simulink model "ex01_model"  (R2023a)
settings: Solver=FixedStepDiscrete  StartTime=0.0  StopTime=20*Ts  RelTol=1e-3
values from neighbouring files (symbols this model uses):
  Fc = 1e3    (= 1000)    [ex00.m]    (also in ex01_config.m; ex02_config.m)
  L = 2    [ex01_config.m]    (also in ex02_config.m = 3)
  Ts = 1/Fs    (= 6.25e-05)    [ex00.m]    (also in ex01_config.m; ex02_config.m)
libraries: dspsrcs4 x1, dspsigops x1
settings Model: Creator=daniele  LastModifiedBy=daniele
settings SolverCC: AlgebraicLoopSolver=TrustRegion
settings DataIOCC: ReturnWorkspaceOutputs=off
settings DebuggingCC: UnconnectedInputMsg=warning  UnconnectedOutputMsg=warning  UnconnectedLineMsg=warning  ArithmeticOperatorsInVariantConditions=warning
settings ModelReferenceCC: EnableRefExpFcnMdlSchedulingChecks=on
settings SFSimCC: CustomCodeUndefinedFunction=UseInterfaceOnly

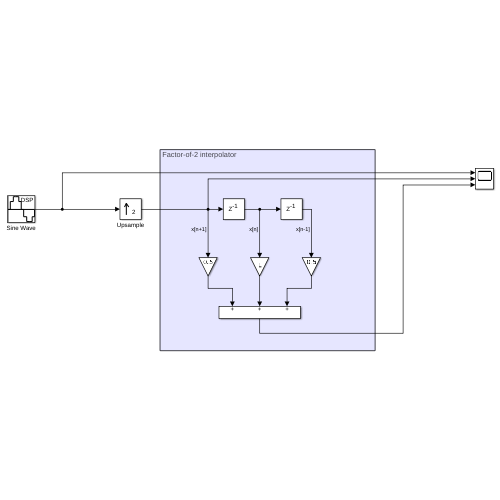
[thumbnail: Simulink's stored preview of the top-level diagram]
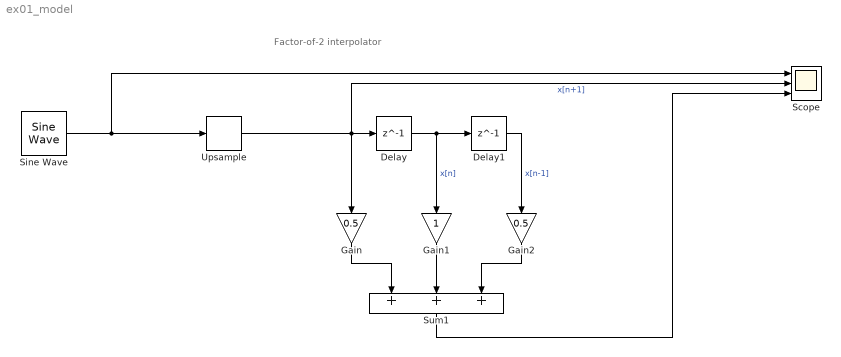
== system ex01_model ==
  note: Factor-of-2 interpolator
  Delay : Delay  DelayLength=1
  Delay1 : Delay  DelayLength=1
  Gain : Gain  Gain=0.5
  Gain1 : Gain
  Gain2 : Gain  Gain=0.5
  Scope : Scope  NumInputPorts=3
  Sine Wave : dspsrcs4/Sine Wave  Amplitude=1  Frequency=Fc  Phase=0  SampleMode=Discrete  OutComplex=Real  CompMethod=Trigonometric fcn  TableSize=Speed  SampleTime=Ts  SamplesPerFrame=1  ResetState=Restart at time zero  OutputFrames=off  dataType=double  wordLen=16  udDataType=sfix(16)  fracBitsMode=Best precision  numFracBits=15  OutDataTypeStr=double  LastOutDataTypeStr=double
  Sum1 : Sum  Inputs=+++
  Upsample : dspsigops/Upsample  FactorSource=Dialog parameter  N=L  Nmax=16  phase=0  RateOptions=Allow multirate processing  ic=0  mode=Unused parameter value
      settings: LibrarySourceBlock=dsphdlsupportsigops/Upsample
  wires:
  Sine Wave/1 -> Upsample/1, Scope/1
  Delay/1 -> Gain1/1, Delay1/1  "x[n]"
  Delay1/1 -> Gain2/1  "x[n-1]"
  Upsample/1 -> Gain/1, Scope/2, Delay/1  "x[n+1]"
  Sum1/1 -> Scope/3
  Gain2/1 -> Sum1/3
  Gain1/1 -> Sum1/2
  Gain/1 -> Sum1/1
